simulink model "player_ball_7_8players3_2"  (R2021b)
settings: Solver=VariableStepAuto  StartTime=0.0  StopTime=300  RelTol=1e-3
model workspace (MAT data in the model file):
  trailfuzzy = 'trailfuzzy.fis'
values from neighbouring files (symbols this model uses):
  initBallPos = fieldCenter    [robotSoccerParams.m]
  robotDetectorMaxHits = 5    [robotSoccerParams.m]
  sampleTime = 0.05    [robotSoccerParams.m]
undefined symbols (not defined in the file or in its folder): DiscIntNeverNeededParam
libraries: mobileRoboticsLib x46, dspindex x15, fuzblock x9
(part 2 of 2)

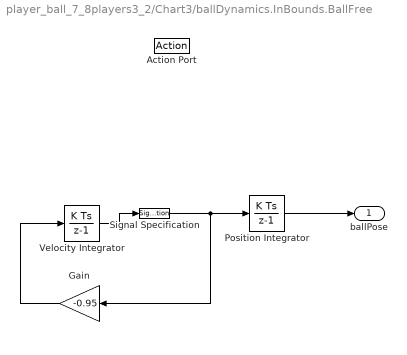
== system player_ball_7_8players3_2/Chart3/ballDynamics.InBounds.BallFree ==
  Action Port : ActionPort
      settings: CopyFcn=Stateflow.SLINSF.SimulinkMan.removeBlockPreDeleteFcn  PreDeleteFcn=Stateflow.SLINSF.SimulinkMan.unsafePredeleteFcn
  Gain : Gain  Gain=-0.95
  Position Integrator : DiscreteIntegrator  InitialCondition=initBallPos  SampleTime=-1  StateName=ballPos  ICPrevOutput=DiscIntNeverNeededParam  ICPrevScaledInput=DiscIntNeverNeededParam
  Signal Specification : SignalSpecification  Dimensions=[1 2]
  Velocity Integrator : DiscreteIntegrator  InitialCondition=[0 0]  SampleTime=-1  StateName=ballVel  ICPrevOutput=DiscIntNeverNeededParam  ICPrevScaledInput=DiscIntNeverNeededParam
  ballPose : Outport  VectorParamsAs1DForOutWhenUnconnected=off
  wires:
  Gain/1 -> Velocity Integrator/1
  Velocity Integrator/1 -> Signal Specification/1
  Position Integrator/1 -> ballPose/1
  Signal Specification/1 -> Position Integrator/1, Gain/1

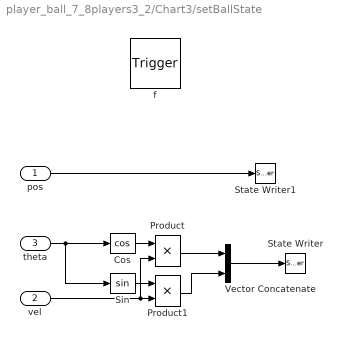
== system player_ball_7_8players3_2/Chart3/setBallState ==
  pos : Inport  OutDataTypeStr=double  PortDimensions=[1 2]
  vel : Inport  Port=2  OutDataTypeStr=double  PortDimensions=1
  theta : Inport  Port=3  OutDataTypeStr=double  PortDimensions=1
  f : TriggerPort  TriggerType=function-call  VariantControl=(inherit)
      settings: CopyFcn=Stateflow.SLINSF.SimulinkMan.removeBlockPreDeleteFcn  PreDeleteFcn=Stateflow.SLINSF.SimulinkMan.unsafePredeleteFcn
  Cos : Trigonometry  Operator=cos
  Product : Product
  Product1 : Product
  Sin : Trigonometry
  State Writer : StateWriter  StateOwnerBlock=../../ballDynamics.InBounds.BallFree/Velocity Integrator  StateName=ballVel
  State Writer1 : StateWriter  StateOwnerBlock=../../ballDynamics.InBounds.BallFree/Position Integrator  StateName=ballPos
  Vector Concatenate : Concatenate  Mode=Multidimensional array  ConcatenateDimension=2
  wires:
  pos/1 -> State Writer1/1
  Vector Concatenate/1 -> State Writer/1
  Cos/1 -> Product/1
  vel/1 -> Product/2, Product1/2
  theta/1 -> Sin/1, Cos/1
  Product/1 -> Vector Concatenate/1
  Product1/1 -> Vector Concatenate/2
  Sin/1 -> Product1/1

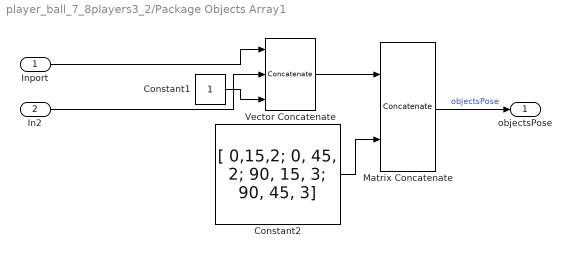
== system player_ball_7_8players3_2/Package Objects Array1 ==
  Inport : Inport
  In2 : Inport  Port=2
  Constant1 : Constant
  Constant2 : Constant  Value=[ 0,15,2; 0, 45, 2; 90, 15, 3; 90, 45, 3]
  Matrix Concatenate : Concatenate  Mode=Multidimensional array
  Vector Concatenate : Concatenate  NumInputs=3  Mode=Multidimensional array  ConcatenateDimension=2
  objectsPose : Outport  VectorParamsAs1DForOutWhenUnconnected=off
  wires:
  In2/1 -> Vector Concatenate/2
  Constant1/1 -> Vector Concatenate/3
  Inport/1 -> Vector Concatenate/1
  Constant2/1 -> Matrix Concatenate/2
  Matrix Concatenate/1 -> objectsPose/1  "objectsPose"
  Vector Concatenate/1 -> Matrix Concatenate/1

== matlab function player_ball_7_8players3_2/Zero Pad Detections2 ==
  data: u input size=[maxHits 3]; y output size=[maxHits 3]; maxHits parameter
function y = zeroPad(u,maxHits)
% Zero-pads object detections to work with arrays of buses

y = zeros(maxHits,3);
numElems = min(size(u,1),maxHits);
for idx = 1:numElems
   y(idx,1:3) = u(idx,1:3); 
end

== matlab function player_ball_7_8players3_2/Plot Soccer Field ==
function plotSoccerField
% Plots the soccer field once the figure window for the environment has
% been initialized

coder.extrinsic('evalin');
persistent hasPlotted
if isempty(hasPlotted)
    evalin('base','plotSoccerField');
    hasPlotted = true;
end

== matlab function player_ball_7_8players3_2/Zero Pad Detections3 ==
  data: u input size=[maxHits 3]; y output size=[maxHits 3]; maxHits parameter
function y = zeroPad(u,maxHits)
% Zero-pads object detections to work with arrays of buses

y = zeros(maxHits,3);
numElems = min(size(u,1),maxHits);
for idx = 1:numElems
   y(idx,1:3) = u(idx,1:3); 
end

== matlab function player_ball_7_8players3_2/ball ==
  data: u input; y output; ballHeld output; robotIdx output; ballHeld input; robotIdx input; aggression output

function [y,ballHeld, robotIdx, aggression]= fcn(u,ballHeld,robotIdx)
a = u(1,:);
b = u(2,:);
c = u(3,:);
d = u(4,:);
e = u(5,:);
robotIdx =1;
aggression = 4;
if a(3) ==1
    y = a;


elseif b(3) ==1
    y = b;


elseif c(3)==1
    y=c;


elseif d(3)==1
    y=d;


else
    y = e;


end
if y(1)  <= 1.1
    ballHeld = 1;
    %robotIdx =1;
    %possession = robotIdx;

else
    ballHeld =0;
    %robotIdx =0;

end

== matlab function player_ball_7_8players3_2/Ball Dynamics ==
  data: ballPose output; ballHeld input; KickPower input; rPose_x input; rPose_y input; rPose_theta input
function ballPose  = fcn(ballHeld, KickPower,rPose_x, rPose_y, rPose_theta)
ballPose = [25 10];
if ballHeld == 1 
    ballPose = [rPose_x rPose_y] + (0.8 + 0.3)*[cos(rPose_theta) sin(rPose_theta)];

elseif KickPower >= 5.5 && ballHeld == 1
    %ballPose = KickPower*[rPose_x rPose_y] + (0.8 + 0.3)*[cos(rPose_theta) sin(rPose_theta)];
    ballHeld = 0
    ballPose = KickPower*[rPose_x rPose_y] + (0.8 + 0.3)*[cos(rPose_theta) sin(rPose_theta)];
    %if KickPower ~=0
    %    ballPose = KickPower*[rPose_x rPose_y] + (0.8 + 0.3)*[cos(rPose_theta) sin(rPose_theta)];
    %end

end

== matlab function player_ball_7_8players3_2/MATLAB Function ==
  data: u input; y output
function y = fcn(u)

if u > 3.15
    u = pi -(u - pi);
end

if u <-3.15
    u = pi + (u + pi);
end     

y = u;

== matlab function player_ball_7_8players3_2/idx3 goal_range_angles ==
  data: u input; goalRight_angle output; goalRange output; goalLeft_angle output; rPose_x input; rPose_y input
% function y = fcn(u)
% for i = 1:5
%     if u(i,3) == 1
%         a = u(i,:)
%     end
% end
% % b = u(2,:)
% % c = u(3,:)
% % d = u(4,:)
% % e = u(5,:)
% y = a;
% end
%two indexes are same. How to identify right and left angles
% for now randomly assigned the values
% goal range is minimum of the two 


function [goalRight_angle,goalRange, goalLeft_angle]= fcn(u,rPose_x, rPose_y)
goalRight_angle=0;
goalLeft_angle=0;
right_range = 0;
left_range =0;

x=0;
%if rPose_y1> 15 &&  rPose_y1< 45 && rPose_theta1 > 0
leftPolePose = [90 45];
rightPolePose = [90 15];
robotPose = [rPose_x rPose_y];
rightPole_dist = norm(rightPolePose - robotPose);
leftPole_dist = norm(leftPolePose - robotPose);
if rightPole_dist< leftPole_dist
    k=0;
    for i= 1:5
        if u(i,3) == 3 && k==0
            goalRight_angle = u(i,2);
            right_range = u(i,1);
            k = k+1;
        elseif u(i,3) ==3 && k==1
            goalLeft_angle = u(i,2);
            left_range = u(i,1);
            k =0;

        end
    end
else
    k=0;
    for i= 1:5
        if u(i,3) == 3 && k==0
            goalLeft_angle = u(i,2);
            left_range = u(i,1);
            k = k+1;
        elseif u(i,3) ==3 && k==1
            goalRight_angle = u(i,2);
            right_range = u(i,1);
            k =0;

        end
    end
end

if right_range < left_range
    goalRange = right_range;
else
    goalRange = left_range;
end

== matlab function player_ball_7_8players3_2/Zero Pad Detections4 ==
  data: u input size=[maxHits 3]; y output size=[maxHits 3]; maxHits parameter
function y = zeroPad(u,maxHits)
% Zero-pads object detections to work with arrays of buses

y = zeros(maxHits,3);
numElems = min(size(u,1),maxHits);
for idx = 1:numElems
   y(idx,1:3) = u(idx,1:3); 
end

== matlab function player_ball_7_8players3_2/Ball Dynamics1 ==
  data: ballPose output; ballHeld input; KickPower input; rPose_x input; rPose_y input; rPose_theta input
function ballPose  = fcn(ballHeld, KickPower,rPose_x, rPose_y, rPose_theta)
ballPose = [25 10];
if ballHeld == 1 
    ballPose = [rPose_x rPose_y] + (0.8 + 0.3)*[cos(rPose_theta) sin(rPose_theta)];

elseif KickPower >= 5.5 && ballHeld == 1
    %ballPose = KickPower*[rPose_x rPose_y] + (0.8 + 0.3)*[cos(rPose_theta) sin(rPose_theta)];
    ballHeld = 0
    ballPose = KickPower*[rPose_x rPose_y] + (0.8 + 0.3)*[cos(rPose_theta) sin(rPose_theta)];
    %if KickPower ~=0
    %    ballPose = KickPower*[rPose_x rPose_y] + (0.8 + 0.3)*[cos(rPose_theta) sin(rPose_theta)];
    %end

end

== matlab function player_ball_7_8players3_2/MATLAB Function1 ==
  data: u input; y output
function y = fcn(u)

if u > 3.15
    u = pi -(u - pi);
end

if u <-3.15
    u = pi + (u + pi);
end     

y = u;

== matlab function player_ball_7_8players3_2/Zero Pad Detections1 ==
  data: u input size=[maxHits 3]; y output size=[maxHits 3]; maxHits parameter
function y = zeroPad(u,maxHits)
% Zero-pads object detections to work with arrays of buses

y = zeros(maxHits,3);
numElems = min(size(u,1),maxHits);
for idx = 1:numElems
   y(idx,1:3) = u(idx,1:3); 
end

== matlab function player_ball_7_8players3_2/Zero Pad Detections5 ==
  data: u input size=[maxHits 3]; y output size=[maxHits 3]; maxHits parameter
function y = zeroPad(u,maxHits)
% Zero-pads object detections to work with arrays of buses

y = zeros(maxHits,3);
numElems = min(size(u,1),maxHits);
for idx = 1:numElems
   y(idx,1:3) = u(idx,1:3); 
end

== matlab function player_ball_7_8players3_2/Zero Pad Detections6 ==
  data: u input size=[maxHits 3]; y output size=[maxHits 3]; maxHits parameter
function y = zeroPad(u,maxHits)
% Zero-pads object detections to work with arrays of buses

y = zeros(maxHits,3);
numElems = min(size(u,1),maxHits);
for idx = 1:numElems
   y(idx,1:3) = u(idx,1:3); 
end

== matlab function player_ball_7_8players3_2/Zero Pad Detections7 ==
  data: u input size=[maxHits 3]; y output size=[maxHits 3]; maxHits parameter
function y = zeroPad(u,maxHits)
% Zero-pads object detections to work with arrays of buses

y = zeros(maxHits,3);
numElems = min(size(u,1),maxHits);
for idx = 1:numElems
   y(idx,1:3) = u(idx,1:3); 
end

== matlab function player_ball_7_8players3_2/ball1 ==
  data: u input; y output; ballHeld output; robotIdx output; ballHeld input; robotIdx input; interception output

function [y,ballHeld, robotIdx, interception]= fcn(u,ballHeld,robotIdx)

a = u(1,:);
b = u(2,:);
c = u(3,:);
d = u(4,:);
e = u(5,:);
robotIdx =2;
interception = 2;
if a(3) ==1
    y = a;


elseif b(3) ==1
    y = b;


elseif c(3)==1
    y=c;


elseif d(3)==1
    y=d;


else
    y = e;


end
if y(1)  <= 1.1
    ballHeld = 1;
    %robotIdx =1;
    %possession = robotIdx;

else
    ballHeld =0;
    %robotIdx =0;

end

== matlab function player_ball_7_8players3_2/idx3 goal_range_angles1 ==
  data: u input; goalRight_angle output; goalRange output; goalLeft_angle output; rPose_x input; rPose_y input
% function y = fcn(u)
% for i = 1:5
%     if u(i,3) == 1
%         a = u(i,:)
%     end
% end
% % b = u(2,:)
% % c = u(3,:)
% % d = u(4,:)
% % e = u(5,:)
% y = a;
% end
%two indexes are same. How to identify right and left angles
% for now randomly assigned the values
% goal range is minimum of the two 


function [goalRight_angle,goalRange, goalLeft_angle]= fcn(u,rPose_x,rPose_y)
goalRight_angle=0;
goalLeft_angle=0;
right_range = 0;
left_range =0;

x=0;
%if rPose_y1> 15 &&  rPose_y1< 45 && rPose_theta1 > 0
leftPolePose = [0 45];
rightPolePose = [0 15];
robotPose = [rPose_x rPose_y];
rightPole_dist = norm(rightPolePose - robotPose);
leftPole_dist = norm(leftPolePose - robotPose);
if rightPole_dist< leftPole_dist
    k=0;
    for i= 1:5
        if u(i,3) == 2 && k==0
            goalRight_angle = u(i,2);
            right_range = u(i,1);
            k = k+1;
        elseif u(i,3) ==2 && k==1
            goalLeft_angle = u(i,2);
            left_range = u(i,1);
            k =0;

        end
    end
else
    k=0;
    for i= 1:5
        if u(i,3) == 2 && k==0
            goalLeft_angle = u(i,2);
            left_range = u(i,1);
            k = k+1;
        elseif u(i,3) ==2 && k==1
            goalRight_angle = u(i,2);
            right_range = u(i,1);
            k =0;

        end
    end
end

if right_range < left_range
    goalRange = right_range;
else
    goalRange = left_range;
end

== matlab function player_ball_7_8players3_2/Zero Pad Detections8 ==
  data: u input size=[maxHits 3]; y output size=[maxHits 3]; maxHits parameter
function y = zeroPad(u,maxHits)
% Zero-pads object detections to work with arrays of buses

y = zeros(maxHits,3);
numElems = min(size(u,1),maxHits);
for idx = 1:numElems
   y(idx,1:3) = u(idx,1:3); 
end

== matlab function player_ball_7_8players3_2/Zero Pad Detections9 ==
  data: u input size=[maxHits 3]; y output size=[maxHits 3]; maxHits parameter
function y = zeroPad(u,maxHits)
% Zero-pads object detections to work with arrays of buses

y = zeros(maxHits,3);
numElems = min(size(u,1),maxHits);
for idx = 1:numElems
   y(idx,1:3) = u(idx,1:3); 
end

== stateflow chart player_ball_7_8players3_2/Chart3 ==
  state ballDynamics [parallel]
    en:
    coder.extrinsic('randn');
    setBallState([45 30],0,0);
    Team1score = 0;
    settings: executionOrder=2
    state InBounds
      en:
      randNum = randn(2,1);
      state BallFree
      state BallHeld
        en,du:
        ballPose = [rPose_X rPose_Y] + ...
        (0.8+0.3)*[cos(rPose_Theta) sin(rPose_Theta)];
      (default) -> BallFree
      BallHeld -> BallFree : [kickPower>2]{setBallState(ballPose,kickPower*3+BallVel, ...
          |  rPose_Theta),possession =0}
      BallFree -> BallHeld : [after(1,sec) && ...
          |  ballheld > 0]
    state Team2
      en:
      Team2score = 0;
      du:
      Team2score = Team2score + 1;
    state Team1
      en:
      Team1score = Team1score + 1;
    state Outofbounds
      en:
      ballPose = [45 30];
      setBallState(ballPose,0,rPose_Theta)
    (default) -> InBounds
    InBounds -> Team2 [order 3] : [ballPose(1) >= 90 && ballPose(2) >=15 && ballPose(2)<=45  ]
    Team2 -> InBounds : [after(1,sec)]
    InBounds -> Team1 [order 2] : [ballPose(1) <= 0 && ballPose(2) >= 15 && ballPose(2) <= 45]
    Team1 -> InBounds : [after(1,sec)]
    Outofbounds -> InBounds : [after(1,sec)]
    InBounds -> Outofbounds [order 1] : [ballPose(1) > 90 || ballPose(2) > 60 || ballPose(1) < 0 || ballPose(2) < 0]
  state Posession [parallel]
    en:
    possession=0;
    ballheld =0;
    du:
    %possession=0;
    for i=1:8
    if ballHeld(i) == 1
    possession = i
    % else
    % possession = 0;
    end
    end
    if possession ~=0
    rPose_X = rPose_x(possession);
    rPose_Y = rPose_y(possession);
    rPose_Theta = rPose_theta(possession);
    kickPower = KickPower(possession);
    BallVel = ballVel(possession);
    ballheld = ballHeld(possession)
    if ballheld == 0
    %   teamHeld = 1;
    % else
    teamHeld = 0
    possession = 0
    end
    if possession == 1 || possession == 2 || possession ==3 || possession == 4
    teamHeld = 1
    elseif possession ==5 || possession == 6 || possession == 7 || possession ==8
    teamHeld = 2
    end
    %else
    %rPose_X= 0;
    %rPose_Y =0;
    %rPose_Theta = 0;
    %kickPower = 0;
    % BallVel = 0;
    % ballheld = 0;
    %teamHeld =0;
    end
    settings: executionOrder=1
  state setBallState(pos,vel,theta) [function]
  data: sf_internal_action_state_placeholder_data local double size=1 =0; pos function_input double size=[1 2]; vel function_input double size=1; theta function_input double size=1; ballHeld input; KickPower input; rPose_x input; rPose_y input; rPose_theta input; robotIdx input; ballPose output; randNum local; action local; ballVel input; i local; possession local; BallVel local; ballheld local; kickPower local; rPose_Theta local; rPose_X local; rPose_Y local; teamHeld output; Team1score output; Team2score output

== matlab function player_ball_7_8players3_2/ball3 ==
  data: u input; y output; ballHeld output; robotIdx output; ballHeld input; robotIdx input

function [y,ballHeld, robotIdx]= fcn(u,ballHeld,robotIdx)
a = u(1,:);
b = u(2,:);
c = u(3,:);
d = u(4,:);
e = u(5,:);
robotIdx =3;
if a(3) ==1
    y = a;


elseif b(3) ==1
    y = b;


elseif c(3)==1
    y=c;


elseif d(3)==1
    y=d;


else
    y = e;


end
if y(1)  <= 1.1
    ballHeld = 1;
    %robotIdx =1;
    %possession = robotIdx;

else
    ballHeld =0;
    %robotIdx =0;

end

== matlab function player_ball_7_8players3_2/idx3 goal_range_angles3 ==
  data: u input; goalRight_angle output; goalRange output; goalLeft_angle output; rPose_x input; rPose_y input
% function y = fcn(u)
% for i = 1:5
%     if u(i,3) == 1
%         a = u(i,:)
%     end
% end
% % b = u(2,:)
% % c = u(3,:)
% % d = u(4,:)
% % e = u(5,:)
% y = a;
% end
%two indexes are same. How to identify right and left angles
% for now randomly assigned the values
% goal range is minimum of the two 


function [goalRight_angle,goalRange, goalLeft_angle]= fcn(u,rPose_x, rPose_y)
goalRight_angle=0;
goalLeft_angle=0;
right_range = 0;
left_range =0;

x=0;
%if rPose_y1> 15 &&  rPose_y1< 45 && rPose_theta1 > 0
leftPolePose = [90 45];
rightPolePose = [90 15];
robotPose = [rPose_x rPose_y];
rightPole_dist = norm(rightPolePose - robotPose);
leftPole_dist = norm(leftPolePose - robotPose);
if rightPole_dist< leftPole_dist
    k=0;
    for i= 1:5
        if u(i,3) == 3 && k==0
            goalRight_angle = u(i,2);
            right_range = u(i,1);
            k = k+1;
        elseif u(i,3) ==3 && k==1
            goalLeft_angle = u(i,2);
            left_range = u(i,1);
            k =0;

        end
    end
else
    k=0;
    for i= 1:5
        if u(i,3) == 3 && k==0
            goalLeft_angle = u(i,2);
            left_range = u(i,1);
            k = k+1;
        elseif u(i,3) ==3 && k==1
            goalRight_angle = u(i,2);
            right_range = u(i,1);
            k =0;

        end
    end
end

if right_range < left_range
    goalRange = right_range;
else
    goalRange = left_range;
end

== matlab function player_ball_7_8players3_2/Zero Pad Detections10 ==
  data: u input size=[maxHits 3]; y output size=[maxHits 3]; maxHits parameter
function y = zeroPad(u,maxHits)
% Zero-pads object detections to work with arrays of buses

y = zeros(maxHits,3);
numElems = min(size(u,1),maxHits);
for idx = 1:numElems
   y(idx,1:3) = u(idx,1:3); 
end

== matlab function player_ball_7_8players3_2/Zero Pad Detections11 ==
  data: u input size=[maxHits 3]; y output size=[maxHits 3]; maxHits parameter
function y = zeroPad(u,maxHits)
% Zero-pads object detections to work with arrays of buses

y = zeros(maxHits,3);
numElems = min(size(u,1),maxHits);
for idx = 1:numElems
   y(idx,1:3) = u(idx,1:3); 
end

== matlab function player_ball_7_8players3_2/Zero Pad Detections12 ==
  data: u input size=[maxHits 3]; y output size=[maxHits 3]; maxHits parameter
function y = zeroPad(u,maxHits)
% Zero-pads object detections to work with arrays of buses

y = zeros(maxHits,3);
numElems = min(size(u,1),maxHits);
for idx = 1:numElems
   y(idx,1:3) = u(idx,1:3); 
end

== matlab function player_ball_7_8players3_2/ball4 ==
  data: u input; y output; ballHeld output; robotIdx output; ballHeld input; robotIdx input

function [y,ballHeld, robotIdx]= fcn(u,ballHeld,robotIdx)
% a = u(1,:);
% b = u(2,:);
% c = u(3,:);
% d = u(4,:);
% e = u(5,:);
% robotIdx =2;
% if a(3) ==1
%     y = a;
% 
% 
% elseif b(3) ==1
%     y = b;
% 
% 
% elseif c(3)==1
%     y=c;
% 
% 
% elseif d(3)==1
%     y=d;
% 
% 
% else
%     y = e;
% 
% 
% end
% if y(1)  <= 1.1
%     ballHeld = 1;
%     %robotIdx =2;
% 
% else
%     ballHeld =0;
%     %robotIdx =0;
% 
% end
a = u(1,:);
b = u(2,:);
c = u(3,:);
d = u(4,:);
e = u(5,:);
robotIdx =4;
if a(3) ==1
    y = a;


elseif b(3) ==1
    y = b;


elseif c(3)==1
    y=c;


elseif d(3)==1
    y=d;


else
    y = e;


end
if y(1)  <= 1.1
    ballHeld = 1;
    %robotIdx =1;
    %possession = robotIdx;

else
    ballHeld =0;
    %robotIdx =0;

end

== matlab function player_ball_7_8players3_2/idx3 goal_range_angles4 ==
  data: u input; goalRight_angle output; goalRange output; goalLeft_angle output; rPose_x input; rPose_y input
% function y = fcn(u)
% for i = 1:5
%     if u(i,3) == 1
%         a = u(i,:)
%     end
% end
% % b = u(2,:)
% % c = u(3,:)
% % d = u(4,:)
% % e = u(5,:)
% y = a;
% end
%two indexes are same. How to identify right and left angles
% for now randomly assigned the values
% goal range is minimum of the two 


function [goalRight_angle,goalRange, goalLeft_angle]= fcn(u,rPose_x,rPose_y)
goalRight_angle=0;
goalLeft_angle=0;
right_range = 0;
left_range =0;

x=0;
%if rPose_y1> 15 &&  rPose_y1< 45 && rPose_theta1 > 0
leftPolePose = [90 45];
rightPolePose = [90 15];
robotPose = [rPose_x rPose_y];
rightPole_dist = norm(rightPolePose - robotPose);
leftPole_dist = norm(leftPolePose - robotPose);
if rightPole_dist< leftPole_dist
    k=0;
    for i= 1:5
        if u(i,3) == 3 && k==0
            goalRight_angle = u(i,2);
            right_range = u(i,1);
            k = k+1;
        elseif u(i,3) ==3 && k==1
            goalLeft_angle = u(i,2);
            left_range = u(i,1);
            k =0;

        end
    end
else
    k=0;
    for i= 1:5
        if u(i,3) == 3 && k==0
            goalLeft_angle = u(i,2);
            left_range = u(i,1);
            k = k+1;
        elseif u(i,3) ==3 && k==1
            goalRight_angle = u(i,2);
            right_range = u(i,1);
            k =0;

        end
    end
end

if right_range < left_range
    goalRange = right_range;
else
    goalRange = left_range;
end

== matlab function player_ball_7_8players3_2/Ball Dynamics2 ==
  data: ballPose output; ballHeld input; KickPower input; rPose_x input; rPose_y input; rPose_theta input
function ballPose  = fcn(ballHeld, KickPower,rPose_x, rPose_y, rPose_theta)
ballPose = [25 10];
if ballHeld == 1 
    ballPose = [rPose_x rPose_y] + (0.8 + 0.3)*[cos(rPose_theta) sin(rPose_theta)];

elseif KickPower >= 5.5 && ballHeld == 1
    %ballPose = KickPower*[rPose_x rPose_y] + (0.8 + 0.3)*[cos(rPose_theta) sin(rPose_theta)];
    ballHeld = 0
    ballPose = KickPower*[rPose_x rPose_y] + (0.8 + 0.3)*[cos(rPose_theta) sin(rPose_theta)];
    %if KickPower ~=0
    %    ballPose = KickPower*[rPose_x rPose_y] + (0.8 + 0.3)*[cos(rPose_theta) sin(rPose_theta)];
    %end

end

== matlab function player_ball_7_8players3_2/Ball Dynamics3 ==
  data: ballPose output; ballHeld input; KickPower input; rPose_x input; rPose_y input; rPose_theta input
function ballPose  = fcn(ballHeld, KickPower,rPose_x, rPose_y, rPose_theta)
ballPose = [25 10];
if ballHeld == 1 
    ballPose = [rPose_x rPose_y] + (0.8 + 0.3)*[cos(rPose_theta) sin(rPose_theta)];

elseif KickPower >= 5.5 && ballHeld == 1
    %ballPose = KickPower*[rPose_x rPose_y] + (0.8 + 0.3)*[cos(rPose_theta) sin(rPose_theta)];
    ballHeld = 0
    ballPose = KickPower*[rPose_x rPose_y] + (0.8 + 0.3)*[cos(rPose_theta) sin(rPose_theta)];
    %if KickPower ~=0
    %    ballPose = KickPower*[rPose_x rPose_y] + (0.8 + 0.3)*[cos(rPose_theta) sin(rPose_theta)];
    %end

end

== matlab function player_ball_7_8players3_2/Ball Dynamics4 ==
  data: ballPose output; ballHeld input; KickPower input; rPose_x input; rPose_y input; rPose_theta input
function ballPose  = fcn(ballHeld, KickPower,rPose_x, rPose_y, rPose_theta)
ballPose = [25 10];
if ballHeld == 1 
    ballPose = [rPose_x rPose_y] + (0.8 + 0.3)*[cos(rPose_theta) sin(rPose_theta)];

elseif KickPower >= 5.5 && ballHeld == 1
    %ballPose = KickPower*[rPose_x rPose_y] + (0.8 + 0.3)*[cos(rPose_theta) sin(rPose_theta)];
    ballHeld = 0
    ballPose = KickPower*[rPose_x rPose_y] + (0.8 + 0.3)*[cos(rPose_theta) sin(rPose_theta)];
    %if KickPower ~=0
    %    ballPose = KickPower*[rPose_x rPose_y] + (0.8 + 0.3)*[cos(rPose_theta) sin(rPose_theta)];
    %end

end

== matlab function player_ball_7_8players3_2/Ball Dynamics5 ==
  data: ballPose output; ballHeld input; KickPower input; rPose_x input; rPose_y input; rPose_theta input
function ballPose  = fcn(ballHeld, KickPower,rPose_x, rPose_y, rPose_theta)
ballPose = [25 10];
if ballHeld == 1 
    ballPose = [rPose_x rPose_y] + (0.8 + 0.3)*[cos(rPose_theta) sin(rPose_theta)];

elseif KickPower >= 5.5 && ballHeld == 1
    %ballPose = KickPower*[rPose_x rPose_y] + (0.8 + 0.3)*[cos(rPose_theta) sin(rPose_theta)];
    ballHeld = 0
    ballPose = KickPower*[rPose_x rPose_y] + (0.8 + 0.3)*[cos(rPose_theta) sin(rPose_theta)];
    %if KickPower ~=0
    %    ballPose = KickPower*[rPose_x rPose_y] + (0.8 + 0.3)*[cos(rPose_theta) sin(rPose_theta)];
    %end

end

== matlab function player_ball_7_8players3_2/Zero Pad Detections13 ==
  data: u input size=[maxHits 3]; y output size=[maxHits 3]; maxHits parameter
function y = zeroPad(u,maxHits)
% Zero-pads object detections to work with arrays of buses

y = zeros(maxHits,3);
numElems = min(size(u,1),maxHits);
for idx = 1:numElems
   y(idx,1:3) = u(idx,1:3); 
end

== matlab function player_ball_7_8players3_2/Zero Pad Detections14 ==
  data: u input size=[maxHits 3]; y output size=[maxHits 3]; maxHits parameter
function y = zeroPad(u,maxHits)
% Zero-pads object detections to work with arrays of buses

y = zeros(maxHits,3);
numElems = min(size(u,1),maxHits);
for idx = 1:numElems
   y(idx,1:3) = u(idx,1:3); 
end

== matlab function player_ball_7_8players3_2/Zero Pad Detections15 ==
  data: u input size=[maxHits 3]; y output size=[maxHits 3]; maxHits parameter
function y = zeroPad(u,maxHits)
% Zero-pads object detections to work with arrays of buses

y = zeros(maxHits,3);
numElems = min(size(u,1),maxHits);
for idx = 1:numElems
   y(idx,1:3) = u(idx,1:3); 
end

== matlab function player_ball_7_8players3_2/ball2 ==
  data: u input; y output; ballHeld output; robotIdx output; ballHeld input; robotIdx input; aggression output

function [y,ballHeld, robotIdx,aggression]= fcn(u,ballHeld,robotIdx)
a = u(1,:);
b = u(2,:);
c = u(3,:);
d = u(4,:);
e = u(5,:);
robotIdx = 5;
aggression = 5;
if a(3) ==1
    y = a;


elseif b(3) ==1
    y = b;


elseif c(3)==1
    y=c;


elseif d(3)==1
    y=d;


else
    y = e;


end
if y(1)  <= 1.1
    ballHeld = 1;
    %robotIdx =1;

else
    ballHeld =0;
    %robotIdx =0;

end

== matlab function player_ball_7_8players3_2/idx3 goal_range_angles2 ==
  data: u input; goalRight_angle output; goalRange output; goalLeft_angle output; rPose_x input; rPose_y input
function [goalRight_angle,goalRange, goalLeft_angle]= fcn(u,rPose_x,rPose_y)
goalRight_angle=0;
goalLeft_angle=0;
right_range = 0;
left_range =0;

x=0;
%if rPose_y1> 15 &&  rPose_y1< 45 && rPose_theta1 > 0
leftPolePose = [0 45];
rightPolePose = [0 15];
robotPose = [rPose_x rPose_y];
rightPole_dist = norm(rightPolePose - robotPose);
leftPole_dist = norm(leftPolePose - robotPose);
if rightPole_dist< leftPole_dist
    k=0;
    for i= 1:5
        if u(i,3) == 2 && k==0
            goalRight_angle = u(i,2);
            right_range = u(i,1);
            k = k+1;
        elseif u(i,3) ==2 && k==1
            goalLeft_angle = u(i,2);
            left_range = u(i,1);
            k =0;

        end
    end
else
    k=0;
    for i= 1:5
        if u(i,3) == 2 && k==0
            goalLeft_angle = u(i,2);
            left_range = u(i,1);
            k = k+1;
        elseif u(i,3) ==2 && k==1
            goalRight_angle = u(i,2);
            right_range = u(i,1);
            k =0;

        end
    end
end

if right_range < left_range
    goalRange = right_range;
else
    goalRange = left_range;
end

== matlab function player_ball_7_8players3_2/Zero Pad Detections16 ==
  data: u input size=[maxHits 3]; y output size=[maxHits 3]; maxHits parameter
function y = zeroPad(u,maxHits)
% Zero-pads object detections to work with arrays of buses

y = zeros(maxHits,3);
numElems = min(size(u,1),maxHits);
for idx = 1:numElems
   y(idx,1:3) = u(idx,1:3); 
end

== matlab function player_ball_7_8players3_2/ball5 ==
  data: u input; y output; ballHeld output; robotIdx output; ballHeld input; robotIdx input; aggression output

function [y,ballHeld, robotIdx,aggression]= fcn(u,ballHeld,robotIdx)
a = u(1,:);
b = u(2,:);
c = u(3,:);
d = u(4,:);
e = u(5,:);
robotIdx = 6;
aggression = 3;
if a(3) ==1
    y = a;


elseif b(3) ==1
    y = b;


elseif c(3)==1
    y=c;


elseif d(3)==1
    y=d;


else
    y = e;


end
if y(1)  <= 1.1
    ballHeld = 1;
    %robotIdx =1;

else
    ballHeld =0;
    %robotIdx =0;

end

== matlab function player_ball_7_8players3_2/idx3 goal_range_angles5 ==
  data: u input; goalRight_angle output; goalRange output; goalLeft_angle output; rPose_x input; rPose_y input
function [goalRight_angle,goalRange, goalLeft_angle]= fcn(u,rPose_x,rPose_y)
goalRight_angle=0;
goalLeft_angle=0;
right_range = 0;
left_range =0;

x=0;
%if rPose_y1> 15 &&  rPose_y1< 45 && rPose_theta1 > 0
leftPolePose = [0 45];
rightPolePose = [0 15];
robotPose = [rPose_x rPose_y];
rightPole_dist = norm(rightPolePose - robotPose);
leftPole_dist = norm(leftPolePose - robotPose);
if rightPole_dist< leftPole_dist
    k=0;
    for i= 1:5
        if u(i,3) == 2 && k==0
            goalRight_angle = u(i,2);
            right_range = u(i,1);
            k = k+1;
        elseif u(i,3) ==2 && k==1
            goalLeft_angle = u(i,2);
            left_range = u(i,1);
            k =0;

        end
    end
else
    k=0;
    for i= 1:5
        if u(i,3) == 2 && k==0
            goalLeft_angle = u(i,2);
            left_range = u(i,1);
            k = k+1;
        elseif u(i,3) ==2 && k==1
            goalRight_angle = u(i,2);
            right_range = u(i,1);
            k =0;

        end
    end
end

if right_range < left_range
    goalRange = right_range;
else
    goalRange = left_range;
end

== matlab function player_ball_7_8players3_2/Ball Dynamics6 ==
  data: ballPose output; ballHeld input; KickPower input; rPose_x input; rPose_y input; rPose_theta input
function ballPose  = fcn(ballHeld, KickPower,rPose_x, rPose_y, rPose_theta)
ballPose = [25 10];
if ballHeld == 1 
    ballPose = [rPose_x rPose_y] + (0.8 + 0.3)*[cos(rPose_theta) sin(rPose_theta)];

elseif KickPower >= 5.5 && ballHeld == 1
    %ballPose = KickPower*[rPose_x rPose_y] + (0.8 + 0.3)*[cos(rPose_theta) sin(rPose_theta)];
    ballHeld = 0
    ballPose = KickPower*[rPose_x rPose_y] + (0.8 + 0.3)*[cos(rPose_theta) sin(rPose_theta)];
    %if KickPower ~=0
    %    ballPose = KickPower*[rPose_x rPose_y] + (0.8 + 0.3)*[cos(rPose_theta) sin(rPose_theta)];
    %end

end

== matlab function player_ball_7_8players3_2/Zero Pad Detections17 ==
  data: u input size=[maxHits 3]; y output size=[maxHits 3]; maxHits parameter
function y = zeroPad(u,maxHits)
% Zero-pads object detections to work with arrays of buses

y = zeros(maxHits,3);
numElems = min(size(u,1),maxHits);
for idx = 1:numElems
   y(idx,1:3) = u(idx,1:3); 
end

== matlab function player_ball_7_8players3_2/Zero Pad Detections18 ==
  data: u input size=[maxHits 3]; y output size=[maxHits 3]; maxHits parameter
function y = zeroPad(u,maxHits)
% Zero-pads object detections to work with arrays of buses

y = zeros(maxHits,3);
numElems = min(size(u,1),maxHits);
for idx = 1:numElems
   y(idx,1:3) = u(idx,1:3); 
end

== matlab function player_ball_7_8players3_2/ball6 ==
  data: u input; y output; ballHeld output; robotIdx output; ballHeld input; robotIdx input; interception output

function [y,ballHeld, robotIdx,interception]= fcn(u,ballHeld,robotIdx)
a = u(1,:);
b = u(2,:);
c = u(3,:);
d = u(4,:);
e = u(5,:);
robotIdx = 7;
interception = 2;
if a(3) ==1
    y = a;


elseif b(3) ==1
    y = b;


elseif c(3)==1
    y=c;


elseif d(3)==1
    y=d;


else
    y = e;


end
if y(1)  <= 1.1
    ballHeld = 1;
    %robotIdx =1;

else
    ballHeld =0;
    %robotIdx =0;

end

== matlab function player_ball_7_8players3_2/idx3 goal_range_angles6 ==
  data: u input; goalRight_angle output; goalRange output; goalLeft_angle output; rPose_x input; rPose_y input
function [goalRight_angle,goalRange, goalLeft_angle]= fcn(u,rPose_x,rPose_y)
goalRight_angle=0;
goalLeft_angle=0;
right_range = 0;
left_range =0;

x=0;
%if rPose_y1> 15 &&  rPose_y1< 45 && rPose_theta1 > 0
leftPolePose = [0 45];
rightPolePose = [0 15];
robotPose = [rPose_x rPose_y];
rightPole_dist = norm(rightPolePose - robotPose);
leftPole_dist = norm(leftPolePose - robotPose);
if rightPole_dist< leftPole_dist
    k=0;
    for i= 1:5
        if u(i,3) == 2 && k==0
            goalRight_angle = u(i,2);
            right_range = u(i,1);
            k = k+1;
        elseif u(i,3) ==2 && k==1
            goalLeft_angle = u(i,2);
            left_range = u(i,1);
            k =0;

        end
    end
else
    k=0;
    for i= 1:5
        if u(i,3) == 2 && k==0
            goalLeft_angle = u(i,2);
            left_range = u(i,1);
            k = k+1;
        elseif u(i,3) ==2 && k==1
            goalRight_angle = u(i,2);
            right_range = u(i,1);
            k =0;

        end
    end
end

if right_range < left_range
    goalRange = right_range;
else
    goalRange = left_range;
end

== matlab function player_ball_7_8players3_2/Zero Pad Detections19 ==
  data: u input size=[maxHits 3]; y output size=[maxHits 3]; maxHits parameter
function y = zeroPad(u,maxHits)
% Zero-pads object detections to work with arrays of buses

y = zeros(maxHits,3);
numElems = min(size(u,1),maxHits);
for idx = 1:numElems
   y(idx,1:3) = u(idx,1:3); 
end

== matlab function player_ball_7_8players3_2/Zero Pad Detections20 ==
  data: u input size=[maxHits 3]; y output size=[maxHits 3]; maxHits parameter
function y = zeroPad(u,maxHits)
% Zero-pads object detections to work with arrays of buses

y = zeros(maxHits,3);
numElems = min(size(u,1),maxHits);
for idx = 1:numElems
   y(idx,1:3) = u(idx,1:3); 
end

== matlab function player_ball_7_8players3_2/Zero Pad Detections21 ==
  data: u input size=[maxHits 3]; y output size=[maxHits 3]; maxHits parameter
function y = zeroPad(u,maxHits)
% Zero-pads object detections to work with arrays of buses

y = zeros(maxHits,3);
numElems = min(size(u,1),maxHits);
for idx = 1:numElems
   y(idx,1:3) = u(idx,1:3); 
end

== matlab function player_ball_7_8players3_2/ball7 ==
  data: u input; y output; ballHeld output; robotIdx output; ballHeld input; robotIdx input

function [y,ballHeld, robotIdx]= fcn(u,ballHeld,robotIdx)
% a = u(1,:);
% b = u(2,:);
% c = u(3,:);
% d = u(4,:);
% e = u(5,:);
% robotIdx =2;
% if a(3) ==1
%     y = a;
% 
% 
% elseif b(3) ==1
%     y = b;
% 
% 
% elseif c(3)==1
%     y=c;
% 
% 
% elseif d(3)==1
%     y=d;
% 
% 
% else
%     y = e;
% 
% 
% end
% if y(1)  <= 1.1
%     ballHeld = 1;
%     %robotIdx =2;
% 
% else
%     ballHeld =0;
%     %robotIdx =0;
% 
% end
a = u(1,:);
b = u(2,:);
c = u(3,:);
d = u(4,:);
e = u(5,:);
robotIdx =8;
if a(3) ==1
    y = a;


elseif b(3) ==1
    y = b;


elseif c(3)==1
    y=c;


elseif d(3)==1
    y=d;


else
    y = e;


end
if y(1)  <= 1.1
    ballHeld = 1;
    %robotIdx =1;
    %possession = robotIdx;

else
    ballHeld =0;
    %robotIdx =0;

end

== matlab function player_ball_7_8players3_2/idx3 goal_range_angles7 ==
  data: u input; goalRight_angle output; goalRange output; goalLeft_angle output; rPose_x input; rPose_y input
% function y = fcn(u)
% for i = 1:5
%     if u(i,3) == 1
%         a = u(i,:)
%     end
% end
% % b = u(2,:)
% % c = u(3,:)
% % d = u(4,:)
% % e = u(5,:)
% y = a;
% end
%two indexes are same. How to identify right and left angles
% for now randomly assigned the values
% goal range is minimum of the two 


function [goalRight_angle,goalRange, goalLeft_angle]= fcn(u,rPose_x,rPose_y)
goalRight_angle=0;
goalLeft_angle=0;
right_range = 0;
left_range =0;

x=0;
%if rPose_y1> 15 &&  rPose_y1< 45 && rPose_theta1 > 0
leftPolePose = [0 45];
rightPolePose = [0 15];
robotPose = [rPose_x rPose_y];
rightPole_dist = norm(rightPolePose - robotPose);
leftPole_dist = norm(leftPolePose - robotPose);
if rightPole_dist< leftPole_dist
    k=0;
    for i= 1:5
        if u(i,3) == 2 && k==0
            goalRight_angle = u(i,2);
            right_range = u(i,1);
            k = k+1;
        elseif u(i,3) ==2 && k==1
            goalLeft_angle = u(i,2);
            left_range = u(i,1);
            k =0;

        end
    end
else
    k=0;
    for i= 1:5
        if u(i,3) == 2 && k==0
            goalLeft_angle = u(i,2);
            left_range = u(i,1);
            k = k+1;
        elseif u(i,3) ==2 && k==1
            goalRight_angle = u(i,2);
            right_range = u(i,1);
            k =0;

        end
    end
end

if right_range < left_range
    goalRange = right_range;
else
    goalRange = left_range;
end

== matlab function player_ball_7_8players3_2/Zero Pad Detections22 ==
  data: u input size=[maxHits 3]; y output size=[maxHits 3]; maxHits parameter
function y = zeroPad(u,maxHits)
% Zero-pads object detections to work with arrays of buses

y = zeros(maxHits,3);
numElems = min(size(u,1),maxHits);
for idx = 1:numElems
   y(idx,1:3) = u(idx,1:3); 
end

== matlab function player_ball_7_8players3_2/Zero Pad Detections23 ==
  data: u input size=[maxHits 3]; y output size=[maxHits 3]; maxHits parameter
function y = zeroPad(u,maxHits)
% Zero-pads object detections to work with arrays of buses

y = zeros(maxHits,3);
numElems = min(size(u,1),maxHits);
for idx = 1:numElems
   y(idx,1:3) = u(idx,1:3); 
end

== matlab function player_ball_7_8players3_2/Zero Pad Detections24 ==
  data: u input size=[maxHits 3]; y output size=[maxHits 3]; maxHits parameter
function y = zeroPad(u,maxHits)
% Zero-pads object detections to work with arrays of buses

y = zeros(maxHits,3);
numElems = min(size(u,1),maxHits);
for idx = 1:numElems
   y(idx,1:3) = u(idx,1:3); 
end

== matlab function player_ball_7_8players3_2/ball8 ==
  data: u input; y output; ballHeld output; robotIdx output; ballHeld input; robotIdx input; interception output

function [y,ballHeld, robotIdx, interception]= fcn(u,ballHeld,robotIdx)
% a = u(1,:);
% b = u(2,:);
% c = u(3,:);
% d = u(4,:);
% e = u(5,:);
% robotIdx =2;
% if a(3) ==1
%     y = a;
% 
% 
% elseif b(3) ==1
%     y = b;
% 
% 
% elseif c(3)==1
%     y=c;
% 
% 
% elseif d(3)==1
%     y=d;
% 
% 
% else
%     y = e;
% 
% 
% end
% if y(1)  <= 1.1
%     ballHeld = 1;
%     %robotIdx =2;
% 
% else
%     ballHeld =0;
%     %robotIdx =0;
% 
% end
a = u(1,:);
b = u(2,:);
c = u(3,:);
d = u(4,:);
e = u(5,:);
robotIdx =2;
interception = 3;
if a(3) ==1
    y = a;


elseif b(3) ==1
    y = b;


elseif c(3)==1
    y=c;


elseif d(3)==1
    y=d;


else
    y = e;


end
if y(1)  <= 1.1
    ballHeld = 1;
    %robotIdx =1;
    %possession = robotIdx;

else
    ballHeld =0;
    %robotIdx =0;

end

== matlab function player_ball_7_8players3_2/idx3 goal_range_angles8 ==
  data: u input; goalRight_angle output; goalRange output; goalLeft_angle output; rPose_x input; rPose_y input
% function y = fcn(u)
% for i = 1:5
%     if u(i,3) == 1
%         a = u(i,:)
%     end
% end
% % b = u(2,:)
% % c = u(3,:)
% % d = u(4,:)
% % e = u(5,:)
% y = a;
% end
%two indexes are same. How to identify right and left angles
% for now randomly assigned the values
% goal range is minimum of the two 


function [goalRight_angle,goalRange, goalLeft_angle]= fcn(u,rPose_x,rPose_y)
goalRight_angle=0;
goalLeft_angle=0;
right_range = 0;
left_range =0;

x=0;
%if rPose_y1> 15 &&  rPose_y1< 45 && rPose_theta1 > 0
leftPolePose = [0 45];
rightPolePose = [0 15];
robotPose = [rPose_x rPose_y];
rightPole_dist = norm(rightPolePose - robotPose);
leftPole_dist = norm(leftPolePose - robotPose);
if rightPole_dist< leftPole_dist
    k=0;
    for i= 1:5
        if u(i,3) == 2 && k==0
            goalRight_angle = u(i,2);
            right_range = u(i,1);
            k = k+1;
        elseif u(i,3) ==2 && k==1
            goalLeft_angle = u(i,2);
            left_range = u(i,1);
            k =0;

        end
    end
else
    k=0;
    for i= 1:5
        if u(i,3) == 2 && k==0
            goalLeft_angle = u(i,2);
            left_range = u(i,1);
            k = k+1;
        elseif u(i,3) ==2 && k==1
            goalRight_angle = u(i,2);
            right_range = u(i,1);
            k =0;

        end
    end
end

if right_range < left_range
    goalRange = right_range;
else
    goalRange = left_range;
end

== matlab function player_ball_7_8players3_2/MATLAB Function2 ==
  data: team1_A input; ballheld output; team2_A input; ballheld input
function ballheld = fcn(team1_A, team2_A, ballheld)
for i= [1:3]
    if ballheld(i) == 1
        if ballheld(i)==1 && ballheld(5)== 1
            if team1_A(i) >= team2_A(1)
                ballheld(5)=0
            else
                ballheld(i)=0
            end
        end
        if ballheld(i)==1 && ballheld(6)== 1
            if team1_A(i) >= team2_A(2)
                ballheld(6)=0
            else
                ballheld(i)=0
            end
        end
        if ballheld(i)==1 && ballheld(7)== 1
            if team1_A(i) >= team2_A(3)
                ballheld(7)=0
            else
                ballheld(i)=0
            end
        end
    end
end
